simulink model "UPSControl"  (R2025b)
settings: Solver=VariableStepAuto  StartTime=0.0  StopTime=10  FixedStep=Ts  RelTol=1e-3
PostLoadFcn:
  | DataCenterParam;
values from neighbouring files (symbols this model uses):
  generator = struct    [GeneratorParam.m]
  lineInductance = 1e-6    (= 1e-06)    [DataCenterParam.m]    (also in GridParam.m)
  lineResistance = 1e-3    (= 0.001)    [DataCenterParam.m]    (also in GridParam.m)
  loadPower = 5e6    (= 5000000)    [DataCenterParam.m]    (also in LVRT.m; RedundancyAnalysis.m = 10000000)
  machine = struct    [GeneratorParam.m]
  powerTau = 0.005    [DataCenterParam.m]
  Ts = 5e-5    (= 5e-05)    [DataCenterParam.m]    (also in GeneratorParam.m)
  utilizationFactor = 0.45    [DataCenterParam.m]    (also in RedundancyAnalysis.m)
undefined symbols (not defined in the file or in its folder): breaker, ctLimitDelayTime, DiscIntNeverNeededParam, ee_sli_rtmsupport, gcbh, grid, rack, ups
libraries: nesl_utility x96, fl_lib x96, eeGeneralControl x84, ee_lib x80, simulink x68, eeTransforms x30, nesl_utility_internal x16, eeSinusoidalMeasurementV2 x13, slpidlib x12, simulink_extras x12, datacenter_lib x5, batteryecm_lib x4
(part 7 of 13)

== system UPSControl/Server Load/UPS Units/Three UPS Parallel/UPS2/DC-Link/BESS ==
  iPFC : Inport
  Vdc : Inport  Port=2
  iChrg : Inport  Port=3
  vPCC : Inport  Port=4
  Brk : Inport  Port=5
  Battery : batteryecm_lib/Battery  Vnom=400 V  prm_dir=simscape.enum.battery.prm_dir.disabled  R1_dis=5e-2 Ohm  R1_ch=1e-3 Ohm  R1=1e-3 Ohm  prm_AH=simscape.enum.battery.prm_AH.infinite  AH=50 A*hr  V1=11.5 V  AH1=25 A*hr  prm_R2=simscape.enum.battery.prm_R2.disabled  R2=2000 Ohm  Tmeas=298.15 K  charge_measurement_port=simscape.enum.battery.enable.yes  prm_dyn=simscape.enum.battery.prm_dyn.off  Rp1=0.005 Ohm  tau1=30 s  Rp2=0.005 Ohm  tau2=30 s  Rp3=0.005 Ohm  tau3=30 s  Rp4=0.005 Ohm  tau4=30 s  Rp5=0.005 Ohm  tau5=30 s  prm_fade=simscape.enum.battery.prm_fade.disabled  N_fade=100  AH_fade=45 A*hr  R1_fade=2.02 Ohm  R1_ch_fade=2.02 Ohm  V1_fade=10.35 V  prm_age=simscape.enum.battery.prm_age.disabled  prm_age_OCV=simscape.enum.battery.prm_age_OCV.OCV  OCV_age=0.9  SOC_age=60  Tmeas_age=298.15 K  delta_time_age_vec=[0] d  temperature_age_vec=[273] K  OCV_scaling_age=2.2134e6  OCV_offset_age=1.632e6  temp_exp_age=0.515833569 V  t_exp_age=0.75  Vnom_T2=12 V  R1_T2=2.2 Ohm  R1_T2_dis=2.2 Ohm  R1_T2_ch=2.2 Ohm  V1_T2=11.4 V  R2_T2=2200 Ohm  Rp1_T2=0.005 Ohm  tau1_T2=30 s  Rp2_T2=0.005 Ohm  tau2_T2=30 s  Rp3_T2=0.005 Ohm  tau3_T2=30 s  Rp4_T2=0.005 Ohm  tau4_T2=30 s  Rp5_T2=0.005 Ohm  tau5_T2=30 s  Tmeas2=273.15 K  thermal_port=simscape.enum.thermaleffects.omit  thermal_mass=30000 J/K  i_specify=on  i_priority=High  i=0 A  i_nominal_specify=off  i_nominal_value=1  i_nominal_unit=A  v_specify=on  v_priority=None  v=400 V  v_nominal_specify=off  v_nominal_value=1  v_nominal_unit=V  charge_specify=on  charge_priority=None  charge=50 A*hr  charge_nominal_specify=off  charge_nominal_value=1  charge_nominal_unit=A*hr  num_cycles_specify=off  num_cycles_priority=High  num_cycles=0  num_cycles_nominal_specify=off  num_cycles_nominal_value=1  num_cycles_nominal_unit=1  temperature_specify=off  temperature_priority=High  temperature=298.15 K  temperature_nominal_specify=off  temperature_nominal_value=1  temperature_nominal_unit=K
      settings: InternalSimscapePortConfiguration="{\"Bottom\":[],\"Left\":[{\"id\":\"p\",\"label\":\"+\",\"type\":\"foundation.electrical.electrical\"},{\"id\":\"q\",\"label\":\"q\",\"type\":\"output\"}],\"Right\":[{\"id\":\"n\",\"label\":\"-\",\"type\":\"foundation.electrical.electrical\"}],\"Top\":[]}"
  Constant : Constant
  Current Sensor : fl_lib/Electrical/Electrical Sensors/Current Sensor
  Current Sensor1 : fl_lib/Electrical/Electrical Sensors/Current Sensor
  DC-DC Converter Controller : Subsystem
  Delay1 : Delay  DelayLength=1  InitialCondition=400
  Delay2 : Delay  DelayLength=1  InitialCondition=400
  Delay3 : Delay  DelayLength=1  InitialCondition=400
  Electrical Reference2 : fl_lib/Electrical/Electrical Elements/Electrical Reference
  PS-Simulink Converter{,1..3} (4 alike) : nesl_utility/PS-Simulink Converter  PhysicalDomain=network_engine_domain  SubClassName=ps_output  LeftPortType=input  RightPortType=output  PseudoPeriodic=off  Frequencies=[]  VectorFormat=inherit  Unit=inherit  AffineConversion=off
  Simscape Component1 : SimscapeComponentBlock  SourceFile=microgridRenewables.biDirectionalConverter  ComponentPath=microgridRenewables.biDirectionalConverter  ComponentVariants="[\"microgridRenewables.biDirectionalConverter\"]"  ComponentVariantNames="[\"biDirectionalConverter\"]"  ClassName=biDirectionalConverter  SchemaVersion=1  efficiency_option=ee.enum.converters.efficiency.constant  efficiency_fixed=100  i_vec=[0, 2, 5] A  efficiency_vec=[90, 95, 98]  iL_specify=off  iL_priority=High  iL=0 A  iL_nominal_specify=off  iL_nominal_value=1  iL_nominal_unit=A  vc_specify=off  vc_priority=High  vc=0 V  vc_nominal_specify=off  vc_nominal_value=1  vc_nominal_unit=V  i1_specify=off  i1_priority=None  i1=0 A  i1_nominal_specify=off  i1_nominal_value=1  i1_nominal_unit=A  i2_specify=off  i2_priority=None  i2=0 A  i2_nominal_specify=off  i2_nominal_value=1  i2_nominal_unit=A  v1_specify=off  v1_priority=None  v1=0 V  v1_nominal_specify=off  v1_nominal_value=1  v1_nominal_unit=V  v2_specify=off  v2_priority=None  v2=0 V  v2_nominal_specify=off  v2_nominal_value=1  v2_nominal_unit=V
      settings: CopyFcn=simscape.sscblock.internal.componentBlockCallback(gcbh,'COPY')  PreCopyFcn=simscape.sscblock.internal.componentBlockCallback(gcbh,'PRECOPY')  PreDeleteFcn=simscape.sscblock.internal.componentBlockCallback(gcbh,'PREDELETE')  InternalSimscapePortConfiguration="{\"Bottom\":[],\"Left\":[{\"id\":\"Iref\",\"label\":\"Iref\",\"type\":\"input\"},{\"id\":\"p1\",\"label\":\"1+\",\"type\":\"foundation.electrical.electrical\"},{\"id\":\"n1\",\"label\":\"1-\",\"type\":\"foundation.electrical.electrical\"}],\"Right\":[{\"id\":\"p2\",\"label\":\"2+\",\"type\":\"foundation.electrical.electrical\"},{\"id\":\"n2\",\"label\":\"2-\",\"type\":\"foundation.electrical.electrical\"}],\"Top\":[]}"
      mask Type: Bi-directional DC-DC Converter
  Voltage Sensor1 : fl_lib/Electrical/Electrical Sensors/Voltage Sensor
  + : PMIOPort  Side=Left
  - : PMIOPort  Port=2  Side=Right
  Ibatt : Outport
  SOC : Outport  Port=2
  IDCDC : Outport  Port=3
  wires:
  iChrg/1 -> DC-DC Converter Controller/5(iCharge)
  Vdc/1 -> DC-DC Converter Controller/2(Vo)
  Delay1/1 -> DC-DC Converter Controller/3(vBatt)
  iPFC/1 -> DC-DC Converter Controller/4(iPFC)
  Constant/1 -> DC-DC Converter Controller/1(Voref)
  PS-Simulink Converter/1 -> Delay2/1
  Delay2/1 -> Ibatt/1, DC-DC Converter Controller/6(iBatt)
  vPCC/1 -> DC-DC Converter Controller/7(vPCC)
  Brk/1 -> DC-DC Converter Controller/8(Breaker)
  PS-Simulink Converter1/1 -> Delay3/1
  Delay3/1 -> SOC/1
  PS-Simulink Converter2/1 -> Delay1/1
  PS-Simulink Converter3/1 -> IDCDC/1
  connections:
  Electrical Reference2/LConn1 -- Simscape Component1/RConn2 -- Voltage Sensor1/RConn2 -- Battery/RConn1
  Battery/LConn1 -- Current Sensor1/RConn2
  PS-Simulink Converter2/LConn1 -- Voltage Sensor1/RConn1
  -/RConn1 -- Simscape Component1/LConn3
  Current Sensor1/LConn1 -- Simscape Component1/RConn1 -- Voltage Sensor1/LConn1
  DC-DC Converter Controller/RConn1 -- Simscape Component1/LConn1
  PS-Simulink Converter/LConn1 -- Current Sensor1/RConn1
  PS-Simulink Converter1/LConn1 -- Battery/LConn2
  Current Sensor/RConn2 -- Simscape Component1/LConn2
  Current Sensor/LConn1 -- +/RConn1
  PS-Simulink Converter3/LConn1 -- Current Sensor/RConn1

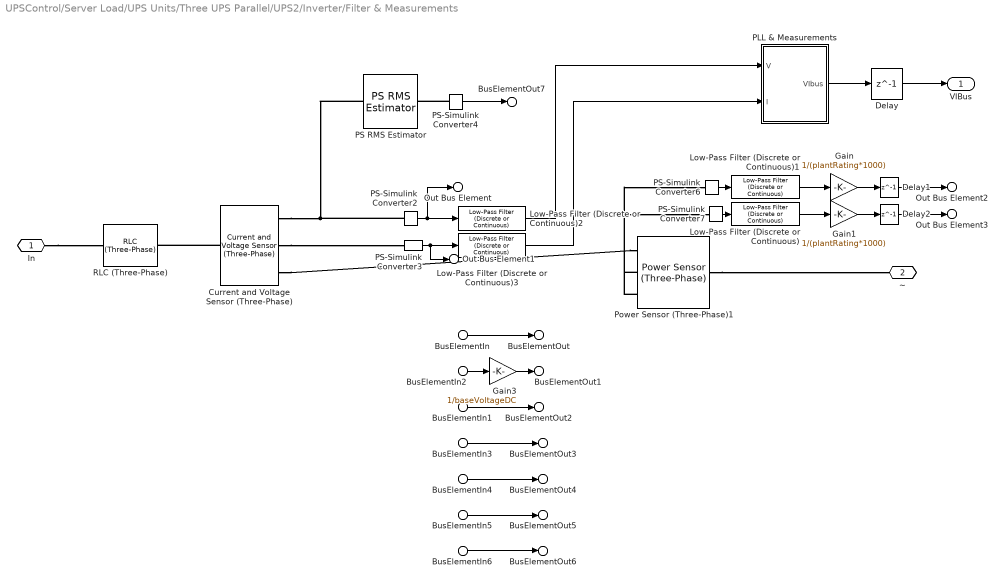
== system UPSControl/Server Load/UPS Units/Three UPS Parallel/UPS2/Inverter/Filter & Measurements ==
  BusElementIn : Inport  PortName=DCBusMeas  Element=SOC
  BusElementIn2 : Inport  PortName=DCBusMeas  Element=Vdc
  BusElementIn1 : Inport  PortName=DCBusMeas  Element=Ibatt
  BusElementIn3 : Inport  PortName=DCBusMeas  Element=Idc
  BusElementIn4 : Inport  PortName=DCBusMeas  Element=ILoad
  BusElementIn5 : Inport  PortName=DCBusMeas  Element=IDCDC
  BusElementIn6 : Inport  PortName=DCBusMeas  Element=UPSBrK
  Current and Voltage Sensor (Three-Phase) : ee_lib/Sensors & Transducers/Current and Voltage Sensor (Three-Phase)  vMeasurementType=ee.enum.vmeasurement.lg  outputUnit=ee.enum.unit.pu  SRated=plantRating*1000 A*V  VRated=Vac V  I_specify=off  I_priority=None  I=[0, 0, 0] A  I_nominal_specify=off  I_nominal_value=1  I_nominal_unit=A  V_specify=off  V_priority=None  V=[0, 0, 0] V  V_nominal_specify=off  V_nominal_value=1  V_nominal_unit=V
      settings: InternalSimscapePortConfiguration="{\"Bottom\":[],\"Left\":[{\"id\":\"N1\",\"label\":\"~1\",\"type\":\"foundation.electrical.three_phase\"}],\"Right\":[{\"id\":\"V_output\",\"label\":\"V\",\"type\":\"output\"},{\"id\":\"I_output\",\"label\":\"I\",\"type\":\"output\"},{\"id\":\"N2\",\"label\":\"~2\",\"type\":\"foundation.electrical.three_phase\"}],\"Top\":[]}"
  Delay : Delay  DelayLength=1
  Delay1 : Delay  DelayLength=1
  Delay2 : Delay  DelayLength=1
  Gain : Gain  Gain=1/(plantRating*1000)
  Gain1 : Gain  Gain=1/(plantRating*1000)
  Gain3 : Gain  Gain=1/baseVoltageDC
  Low-Pass Filter (Discrete or Continuous) : eeGeneralControl/Low-Pass Filter (Discrete or Continuous)  K=1  T=powerTau  B=inf  A=-inf  init_option=Inherited from block input  x0=0  Ts=Ts
  Low-Pass Filter (Discrete or Continuous)1 : eeGeneralControl/Low-Pass Filter (Discrete or Continuous)  K=1  T=powerTau  B=inf  A=-inf  init_option=Inherited from block input  x0=0  Ts=Ts
  Low-Pass Filter (Discrete or Continuous)2 : eeGeneralControl/Low-Pass Filter (Discrete or Continuous)  K=1  T=powerTau/10  B=inf  A=-inf  init_option=Inherited from block input  x0=0  Ts=Ts
  Low-Pass Filter (Discrete or Continuous)3 : eeGeneralControl/Low-Pass Filter (Discrete or Continuous)  K=1  T=powerTau/10  B=inf  A=-inf  init_option=Inherited from block input  x0=0  Ts=Ts
  PLL & Measurements : Subsystem
      mask Display: image('PLL_9_7_2_20_1.png');
  PS RMS Estimator : fl_lib/Physical Signals/Periodic Operators/PS RMS Estimator  f0=60 Hz
      settings: InternalSimscapePortConfiguration="{\"Bottom\":[],\"Left\":[{\"id\":\"I\",\"label\":\"\",\"type\":\"input\"}],\"Right\":[{\"id\":\"O\",\"label\":\"\",\"type\":\"output\"}],\"Top\":[]}"
  PS-Simulink Converter2 : nesl_utility_internal/PS-Simulink Converter  PhysicalDomain=network_engine_domain  SubClassName=ps_output  LeftPortType=input  RightPortType=output  PseudoPeriodic=off  Frequencies=[]  VectorFormat=1-D array  Unit=V  AffineConversion=off
  PS-Simulink Converter3 : nesl_utility_internal/PS-Simulink Converter  PhysicalDomain=network_engine_domain  SubClassName=ps_output  LeftPortType=input  RightPortType=output  PseudoPeriodic=off  Frequencies=[]  VectorFormat=1-D array  Unit=A  AffineConversion=off
  PS-Simulink Converter4 : nesl_utility/PS-Simulink Converter  PhysicalDomain=network_engine_domain  SubClassName=ps_output  LeftPortType=input  RightPortType=output  PseudoPeriodic=off  Frequencies=[]  VectorFormat=inherit  Unit=inherit  AffineConversion=off
  PS-Simulink Converter6 : nesl_utility_internal/PS-Simulink Converter  PhysicalDomain=network_engine_domain  SubClassName=ps_output  LeftPortType=input  RightPortType=output  PseudoPeriodic=off  Frequencies=[]  VectorFormat=1-D array  Unit=W  AffineConversion=off
  PS-Simulink Converter7 : nesl_utility_internal/PS-Simulink Converter  PhysicalDomain=network_engine_domain  SubClassName=ps_output  LeftPortType=input  RightPortType=output  PseudoPeriodic=off  Frequencies=[]  VectorFormat=1-D array  Unit=V*A  AffineConversion=off
  Power Sensor (Three-Phase)1 : ee_lib/Sensors & Transducers/Power Sensor (Three-Phase)  load_type=ee.enum.passive.type_balanced.balanced  f0=60 Hz
      settings: InternalSimscapePortConfiguration="{\"Bottom\":[],\"Left\":[{\"id\":\"N1\",\"label\":\"~1\",\"type\":\"foundation.electrical.three_phase\"}],\"Right\":[{\"id\":\"N2\",\"label\":\"~2\",\"type\":\"foundation.electrical.three_phase\"}],\"Top\":[{\"id\":\"Pm\",\"label\":\"P\",\"type\":\"output\"},{\"id\":\"Qm\",\"label\":\"Q\",\"type\":\"output\"}]}"
  RLC (Three-Phase) : ee_lib/Passive/RLC Assemblies/RLC (Three-Phase)  port_option=ee.enum.threePhasePort.composite  component_structure=ee.enum.rlc.structure.SeriesRL  R=filterResistance %5e-5 Ohm  L=filterInductance%0.00012 H  C=1e-6 F  R_parasitic=0 Ohm  G_parasitic=0 1/Ohm  IL_specify=on  IL_priority=None  IL=[0, 0, 0] A  IL_nominal_specify=off  IL_nominal_value=1  IL_nominal_unit=A  VC_specify=off  VC_priority=High  VC=[0, 0, 0] V  VC_nominal_specify=off  VC_nominal_value=1  VC_nominal_unit=V
      settings: InternalSimscapePortConfiguration="{\"Bottom\":[],\"Left\":[{\"id\":\"N1\",\"label\":\"~1\",\"type\":\"foundation.electrical.three_phase\"}],\"Right\":[{\"id\":\"N2\",\"label\":\"~2\",\"type\":\"foundation.electrical.three_phase\"}],\"Top\":[]}"
  In : PMIOPort  Side=Left
  ~ : PMIOPort  Port=2  Side=Right
  VIBus : Outport
  Out Bus Element : Outport  Port=2  PortName=Meas  Element=voltage
  Out Bus Element1 : Outport  Port=2  PortName=Meas  Element=current
  Out Bus Element2 : Outport  Port=2  PortName=Meas  Element=activePower
  Out Bus Element3 : Outport  Port=2  PortName=Meas  Element=reactivePower
  BusElementOut : Outport  Port=2  PortName=Meas  Element=SOC
  BusElementOut1 : Outport  Port=2  PortName=Meas  Element=Vdc
  BusElementOut2 : Outport  Port=2  PortName=Meas  Element=IBatt
  BusElementOut3 : Outport  Port=2  PortName=Meas  Element=Idc
  BusElementOut4 : Outport  Port=2  PortName=Meas  Element=ILoad
  BusElementOut5 : Outport  Port=2  PortName=Meas  Element=IDCDC
  BusElementOut6 : Outport  Port=2  PortName=Meas  Element=UPSBrK
  BusElementOut7 : Outport  Port=2  PortName=Meas  Element=rmsVoltage
  wires:
  BusElementIn/1 -> BusElementOut/1
  Gain1/1 -> Delay2/1
  Gain/1 -> Delay1/1
  PS-Simulink Converter2/1 -> Out Bus Element/1, Low-Pass Filter (Discrete or Continuous)2/1
  PS-Simulink Converter6/1 -> Low-Pass Filter (Discrete or Continuous)1/1
  PS-Simulink Converter7/1 -> Low-Pass Filter (Discrete or Continuous)/1
  PS-Simulink Converter3/1 -> Out Bus Element1/1, Low-Pass Filter (Discrete or Continuous)3/1
  Low-Pass Filter (Discrete or Continuous)/1 -> Gain1/1
  Low-Pass Filter (Discrete or Continuous)1/1 -> Gain/1
  PLL & Measurements/1(VIbus) -> Delay/1
  Delay/1 -> VIBus/1
  BusElementIn2/1 -> Gain3/1
  Delay1/1 -> Out Bus Element2/1
  Delay2/1 -> Out Bus Element3/1
  BusElementIn1/1 -> BusElementOut2/1
  Gain3/1 -> BusElementOut1/1
  BusElementIn3/1 -> BusElementOut3/1
  BusElementIn4/1 -> BusElementOut4/1
  Low-Pass Filter (Discrete or Continuous)2/1 -> PLL & Measurements/1(V)
  Low-Pass Filter (Discrete or Continuous)3/1 -> PLL & Measurements/2(I)
  BusElementIn5/1 -> BusElementOut5/1
  BusElementIn6/1 -> BusElementOut6/1
  PS-Simulink Converter4/1 -> BusElementOut7/1
  connections:
  Current and Voltage Sensor (Three-Phase)/RConn3 -- Power Sensor (Three-Phase)1/LConn1
  PS-Simulink Converter2/LConn1 -- Current and Voltage Sensor (Three-Phase)/RConn1 -- PS RMS Estimator/LConn1
  Current and Voltage Sensor (Three-Phase)/RConn2 -- PS-Simulink Converter3/LConn1
  Power Sensor (Three-Phase)1/LConn2 -- PS-Simulink Converter6/LConn1
  Power Sensor (Three-Phase)1/LConn3 -- PS-Simulink Converter7/LConn1
  Current and Voltage Sensor (Three-Phase)/LConn1 -- RLC (Three-Phase)/RConn1
  Power Sensor (Three-Phase)1/RConn1 -- ~/RConn1
  In/RConn1 -- RLC (Three-Phase)/LConn1
  PS-Simulink Converter4/LConn1 -- PS RMS Estimator/RConn1

== system UPSControl/Server Load/UPS Units/Three UPS Parallel/UPS2/Inverter/Inverter Controller ==
  VI : Inport
  Power : Inport  Port=2
  Current Limiter : Subsystem
  Droop Control : Subsystem  VariantControl=droop
  VoltageCurrentControl : Subsystem
  mabc : Outport
  wires:
  VI/1 -> VoltageCurrentControl/1(measure), Current Limiter/1(VI)
  VoltageCurrentControl/1(mabc) -> mabc/1
  Droop Control/2(Vqref) -> Current Limiter/3(Vq)
  Droop Control/1(Vdref) -> Current Limiter/2(Vd)
  Droop Control/3(omega) -> VoltageCurrentControl/6(w)
  Droop Control/4(Theta) -> VoltageCurrentControl/7(Angle)
  Current Limiter/3(Idmax) -> VoltageCurrentControl/4(Idmax)
  Current Limiter/2(VqRef) -> VoltageCurrentControl/3(Vqref)
  Current Limiter/1(VdRef) -> VoltageCurrentControl/2(Vdref)
  Current Limiter/4(Iqmax) -> VoltageCurrentControl/5(Iqmax)
  Power/1 -> Droop Control/1(Power)

== system UPSControl/Server Load/UPS Units/Three UPS Parallel/UPS2/Rectifier/Circuit Breaker ==
  BRK : Inport
  Data Type Conversion : DataTypeConversion  OutDataTypeStr=double  SaturateOnIntegerOverflow=off  RndMeth=Floor
  Open Resistance : Gain  Gain=5e7
  Phase Splitter : ee_lib/Connectors & References/Phase Splitter
  Phase Splitter1 : ee_lib/Connectors & References/Phase Splitter
  Simulink-PS Converter : nesl_utility/Simulink-PS Converter  PhysicalDomain=network_engine_domain  SubClassName=ps_input  LeftPortType=input  RightPortType=output  PseudoPeriodic=off  Frequencies=[]  NoiseDistribution=none  NoiseParameters=[]  Unit=1  AffineConversion=off  FilteringAndDerivatives=provide  SimscapeFilterOrder=1  InputFilterTimeConstant=0.001  UdotUserProvided=0
  Variable Resistor : fl_lib/Electrical/Electrical Elements/Variable Resistor  Rmin=1e-3 Ohm  thermalEnable=false  thermal_mass=1 J/K  i_specify=on  i_priority=None  i=0 A  i_nominal_specify=off  i_nominal_value=1  i_nominal_unit=A  v_specify=off  v_priority=None  v=0 V  v_nominal_specify=off  v_nominal_value=1  v_nominal_unit=V  T_specify=off  T_priority=None  T=300 K  T_nominal_specify=off  T_nominal_value=1  T_nominal_unit=K
  Variable Resistor1 : fl_lib/Electrical/Electrical Elements/Variable Resistor  Rmin=1e-3 Ohm  thermalEnable=false  thermal_mass=1 J/K  i_specify=on  i_priority=None  i=0 A  i_nominal_specify=off  i_nominal_value=1  i_nominal_unit=A  v_specify=off  v_priority=None  v=0 V  v_nominal_specify=off  v_nominal_value=1  v_nominal_unit=V  T_specify=off  T_priority=None  T=300 K  T_nominal_specify=off  T_nominal_value=1  T_nominal_unit=K
  Variable Resistor2 : fl_lib/Electrical/Electrical Elements/Variable Resistor  Rmin=1e-3 Ohm  thermalEnable=false  thermal_mass=1 J/K  i_specify=on  i_priority=None  i=0 A  i_nominal_specify=off  i_nominal_value=1  i_nominal_unit=A  v_specify=off  v_priority=None  v=0 V  v_nominal_specify=off  v_nominal_value=1  v_nominal_unit=V  T_specify=off  T_priority=None  T=300 K  T_nominal_specify=off  T_nominal_value=1  T_nominal_unit=K
  ABC2 : PMIOPort  Side=Left
  ~ : PMIOPort  Port=2  Side=Right
  wires:
  Data Type Conversion/1 -> Open Resistance/1
  BRK/1 -> Data Type Conversion/1
  Open Resistance/1 -> Simulink-PS Converter/1
  connections:
  Phase Splitter1/RConn2 -- Variable Resistor1/RConn1
  Variable Resistor1/LConn2 -- Phase Splitter/RConn2
  Phase Splitter1/RConn3 -- Variable Resistor2/RConn1
  Phase Splitter/RConn1 -- Variable Resistor/LConn2
  Variable Resistor2/LConn2 -- Phase Splitter/RConn3
  Phase Splitter1/RConn1 -- Variable Resistor/RConn1
  Phase Splitter1/LConn1 -- ~/RConn1
  Variable Resistor/LConn1 -- Simulink-PS Converter/RConn1 -- Variable Resistor2/LConn1 -- Variable Resistor1/LConn1
  Phase Splitter/LConn1 -- ABC2/RConn1

== system UPSControl/Server Load/UPS Units/Three UPS Parallel/UPS2/Rectifier/Filter & AC measurements ==
  Current : Subsystem
  Current and Voltage Sensor (Three-Phase) : ee_lib/Sensors & Transducers/Current and Voltage Sensor (Three-Phase)  vMeasurementType=ee.enum.vmeasurement.lg  outputUnit=ee.enum.unit.pu  SRated=plantRating*1000 A*V  VRated=Vac V  I_specify=off  I_priority=None  I=[0, 0, 0] A  I_nominal_specify=off  I_nominal_value=1  I_nominal_unit=A  V_specify=off  V_priority=None  V=[0, 0, 0] V  V_nominal_specify=off  V_nominal_value=1  V_nominal_unit=V
      settings: InternalSimscapePortConfiguration="{\"Bottom\":[],\"Left\":[{\"id\":\"N1\",\"label\":\"~1\",\"type\":\"foundation.electrical.three_phase\"}],\"Right\":[{\"id\":\"V_output\",\"label\":\"V\",\"type\":\"output\"},{\"id\":\"I_output\",\"label\":\"I\",\"type\":\"output\"},{\"id\":\"N2\",\"label\":\"~2\",\"type\":\"foundation.electrical.three_phase\"}],\"Top\":[]}"
  Gain : Gain  Gain=1/(plantRating*1000)
  Gain1 : Gain  Gain=1/(plantRating*1000)
  Low-Pass Filter (Discrete or Continuous)1 : eeGeneralControl/Low-Pass Filter (Discrete or Continuous)  K=1  T=10e-3  B=inf  A=-inf  init_option=Inherited from block input  x0=0  Ts=-1
  Low-Pass Filter (Discrete or Continuous)2 : eeGeneralControl/Low-Pass Filter (Discrete or Continuous)  K=1  T=10e-3  B=inf  A=-inf  init_option=Inherited from block input  x0=0  Ts=-1
  PLL : Subsystem
      settings: PortSchema="{\"entries\":[{\"content\":{\"sides\":[{\"content\":{\"connectorIds\":[\"Out1\",\"Out2\",\"Out3\"]},\"type\":\"ConnectorPlacement.EquallySpacedRectSide\",\"uuid\":\"76485780-20fe-4fcf-8224-69648da6ed2a\"},{\"content\":{\"connectorIds\":[\"In1\",\"In2\"],\"side\":\"RIGHT\"},\"type\":\"ConnectorPlacement.EquallySpacedRectSide\",\"uuid\":\"f19a6390-e634-42c7-8d46-4cd80cbab182\"},{\"content\":{\"side\":\"TOP\"},\"type\":\"ConnectorPlacement.EquallySpacedRectSide\",\"uuid\":\"87682f72-1844-428e-be70-ad7ca3191ee3\"}]},\"type\":\"ConnectorPlacement.EquallySpacedConnector\",\"uuid\":\"f2136b07-48ec-402b-adb3-18c0bac2157c\"}],\"packageUris\":[\"http://schema.mathworks.com/mf0/Connector/R2020b\"],\"version\":\"1.0\"}"
  PS-Simulink Converter : nesl_utility/PS-Simulink Converter  PhysicalDomain=network_engine_domain  SubClassName=ps_output  LeftPortType=input  RightPortType=output  PseudoPeriodic=off  Frequencies=[]  VectorFormat=1-D array  Unit=inherit  AffineConversion=off
  PS-Simulink Converter1 : nesl_utility/PS-Simulink Converter  PhysicalDomain=network_engine_domain  SubClassName=ps_output  LeftPortType=input  RightPortType=output  PseudoPeriodic=off  Frequencies=[]  VectorFormat=1-D array  Unit=inherit  AffineConversion=off
  PS-Simulink Converter2 : nesl_utility/PS-Simulink Converter  PhysicalDomain=network_engine_domain  SubClassName=ps_output  LeftPortType=input  RightPortType=output  PseudoPeriodic=off  Frequencies=[]  VectorFormat=inherit  Unit=inherit  AffineConversion=off
  PS-Simulink Converter3 : nesl_utility/PS-Simulink Converter  PhysicalDomain=network_engine_domain  SubClassName=ps_output  LeftPortType=input  RightPortType=output  PseudoPeriodic=off  Frequencies=[]  VectorFormat=inherit  Unit=inherit  AffineConversion=off
  Power Sensor : ee_lib/Sensors & Transducers/Power Sensor (Three-Phase)  load_type=ee.enum.passive.type_balanced.balanced  f0=60 Hz
      settings: InternalSimscapePortConfiguration="{\"Bottom\":[],\"Left\":[{\"id\":\"N1\",\"label\":\"~1\",\"type\":\"foundation.electrical.three_phase\"}],\"Right\":[{\"id\":\"N2\",\"label\":\"~2\",\"type\":\"foundation.electrical.three_phase\"}],\"Top\":[{\"id\":\"Pm\",\"label\":\"P\",\"type\":\"output\"},{\"id\":\"Qm\",\"label\":\"Q\",\"type\":\"output\"}]}"
  RL filter : ee_lib/Passive/RLC Assemblies/RLC (Three-Phase)  port_option=ee.enum.threePhasePort.composite  component_structure=ee.enum.rlc.structure.SeriesRL  R=filterResistanceAFE%0.04 Ohm  L=filterInductanceAFE%6.25e-5 H  C=1e-6 F  R_parasitic=1e-6 Ohm  G_parasitic=1e-6 1/Ohm  IL_specify=on  IL_priority=None  IL=[0, 0, 0] A  IL_nominal_specify=off  IL_nominal_value=1  IL_nominal_unit=A  VC_specify=on  VC_priority=High  VC=[0, 0, 0] V  VC_nominal_specify=off  VC_nominal_value=1  VC_nominal_unit=V
      settings: InternalSimscapePortConfiguration="{\"Bottom\":[],\"Left\":[{\"id\":\"N1\",\"label\":\"~1\",\"type\":\"foundation.electrical.three_phase\"}],\"Right\":[{\"id\":\"N2\",\"label\":\"~2\",\"type\":\"foundation.electrical.three_phase\"}],\"Top\":[]}"
  Voltage : Subsystem
  ABC : PMIOPort  Side=Left
  ABC2 : PMIOPort  Port=2  Side=Right
  Vabc : Outport
  Iabc : Outport  Port=2
  P : Outport  Port=3
  Q : Outport  Port=4
  Id : Outport  Port=5
  freq : Outport  Port=6
  mag : Outport  Port=7
  wires:
  PS-Simulink Converter/1 -> Current/1(Isabc)
  Current/1(Iabc) -> Iabc/1, PLL/1(Iabc)
  PS-Simulink Converter1/1 -> Voltage/1(Vsabc)
  Voltage/1(Vabc) -> Vabc/1, PLL/2(V)
  PS-Simulink Converter2/1 -> Gain/1
  PS-Simulink Converter3/1 -> Gain1/1
  Gain/1 -> Low-Pass Filter (Discrete or Continuous)1/1
  Gain1/1 -> Low-Pass Filter (Discrete or Continuous)2/1
  PLL/1(Id) -> Id/1
  PLL/3(mag) -> mag/1
  PLL/2(freq) -> freq/1
  Low-Pass Filter (Discrete or Continuous)1/1 -> P/1
  Low-Pass Filter (Discrete or Continuous)2/1 -> Q/1
  connections:
  PS-Simulink Converter/LConn1 -- Current and Voltage Sensor (Three-Phase)/RConn2
  PS-Simulink Converter1/LConn1 -- Current and Voltage Sensor (Three-Phase)/RConn1
  Current and Voltage Sensor (Three-Phase)/LConn1 -- ABC/RConn1
  Power Sensor/RConn1 -- RL filter/LConn1
  Power Sensor/LConn1 -- Current and Voltage Sensor (Three-Phase)/RConn3
  PS-Simulink Converter2/LConn1 -- Power Sensor/LConn2
  PS-Simulink Converter3/LConn1 -- Power Sensor/LConn3
  RL filter/RConn1 -- ABC2/RConn1

== system UPSControl/Server Load/UPS Units/Three UPS Parallel/UPS2/Rectifier/PFC Rectifier Controller ==
  VdcRef (V) : Inport
  QRef (pu) : Inport  Port=2
  VdcSens (V) : Inport  Port=3
  VabcSens (pu) : Inport  Port=4
  IabcSens (pu) : Inport  Port=5
  Reset : Inport  Port=6
  Current Controller : Subsystem
  DC Voltage Controller and Current Reference : Subsystem
  PLL : Subsystem
      settings: PortSchema="{\"entries\":[{\"content\":{\"sides\":[{\"content\":{\"connectorIds\":[\"Out1\",\"Out2\",\"Out3\",\"Out4\"]},\"type\":\"ConnectorPlacement.EquallySpacedRectSide\",\"uuid\":\"76485780-20fe-4fcf-8224-69648da6ed2a\"},{\"content\":{\"connectorIds\":[\"In1\"],\"side\":\"RIGHT\"},\"type\":\"ConnectorPlacement.EquallySpacedRectSide\",\"uuid\":\"f19a6390-e634-42c7-8d46-4cd80cbab182\"},{\"content\":{\"side\":\"TOP\"},\"type\":\"ConnectorPlacement.EquallySpacedRectSide\",\"uuid\":\"87682f72-1844-428e-be70-ad7ca3191ee3\"}]},\"type\":\"ConnectorPlacement.EquallySpacedConnector\",\"uuid\":\"f2136b07-48ec-402b-adb3-18c0bac2157c\"}],\"packageUris\":[\"http://schema.mathworks.com/mf0/Connector/R2020b\"],\"version\":\"1.0\"}"
  Rate Transition : RateTransition
  VabcRef (pu) : Outport
  Out Bus Element : Outport  Port=2  PortName=Visualization  Element=pllAngle [rad]
  Out Bus Element1 : Outport  Port=2  PortName=Visualization  Element=pllVmag [pu]
  Out Bus Element2 : Outport  Port=2  PortName=Visualization  Element=Idref [pu]
  Out Bus Element3 : Outport  Port=2  PortName=Visualization  Element=Iqref [pu]
  Out Bus Element5 : Outport  Port=2  PortName=Visualization  Element=IdCntrlError [pu]
  Out Bus Element6 : Outport  Port=2  PortName=Visualization  Element=IqCntrlError [pu]
  wires:
  Current Controller/3(IqCntrlError) -> Out Bus Element6/1
  Current Controller/2(IdCntrlError) -> Out Bus Element5/1
  PLL/1(theta) -> Out Bus Element/1, Current Controller/3(theta)
  Rate Transition/1 -> PLL/1(V)
  DC Voltage Controller and Current Reference/2(iqRef) -> Out Bus Element3/1, Current Controller/2(iqRef)
  DC Voltage Controller and Current Reference/1(idRef) -> Out Bus Element2/1, Current Controller/1(idRef)
  IabcSens (pu)/1 -> Current Controller/6(iabc(PU))
  PLL/3(Vq) -> Current Controller/5(vq)
  PLL/2(Vd) -> Current Controller/4(vd)
  VdcSens (V)/1 -> DC Voltage Controller and Current Reference/4(VdcSens)
  Current Controller/1(vabcRef) -> VabcRef (pu)/1
  PLL/4(mag) -> DC Voltage Controller and Current Reference/2(vPeak), Out Bus Element1/1
  QRef (pu)/1 -> DC Voltage Controller and Current Reference/1(qRef)
  VabcSens (pu)/1 -> Rate Transition/1
  VdcRef (V)/1 -> DC Voltage Controller and Current Reference/3(vdcRef)
  Reset/1 -> Current Controller/7(Reset), DC Voltage Controller and Current Reference/5(Reset)

== system UPSControl/Server Load/UPS Units/Three UPS Parallel/UPS2/Rectifier/Subsystem ==
  In : Inport
  Constant : Constant  Value=0  OutDataTypeStr=boolean
  Delay : Delay  DelayLength=700  SampleTime=ups.sampleTime
  Detect Decrease : simulink/Logic and Bit Operations/Detect Decrease  vinit=0.0  OutDataTypeStr=boolean
  S-R Flip-Flop1 : simulink_extras/Flip Flops/S-R Flip-Flop  initial_condition=0
  Switch : Switch  Criteria=u2 > Threshold  SaturateOnIntegerOverflow=off  InputSameDT=off
  Out : Outport
  wires:
  In/1 -> Detect Decrease/1, Switch/3, Delay/1
  Switch/1 -> Out/1
  Detect Decrease/1 -> S-R Flip-Flop1/1
  Delay/1 -> Switch/1
  S-R Flip-Flop1/1 -> Switch/2
  Constant/1 -> S-R Flip-Flop1/2

== system UPSControl/Server Load/UPS Units/Three UPS Parallel/UPS2/Rectifier/Transfer Control ==
  IBatt : Inport
  Id : Inport  Port=2
  Freq : Inport  Port=3
  Mag : Inport  Port=4
  AND2 : Logic  IconShape=distinctive  AllPortsSameDT=off  OutDataTypeStr=boolean
  AND3 : Logic  IconShape=distinctive  AllPortsSameDT=off  OutDataTypeStr=boolean
  Battery Current Flag : Subsystem
  Data Type Conversion : DataTypeConversion  OutDataTypeStr=boolean  SaturateOnIntegerOverflow=off  RndMeth=Floor
  Frequency Flag : Subsystem
  NOT1 : Logic  Operator=NOT  IconShape=distinctive  AllPortsSameDT=off  OutDataTypeStr=boolean
  NOT2 : Logic  Operator=NOT  IconShape=distinctive  AllPortsSameDT=off  OutDataTypeStr=boolean
  OR : Logic  Operator=OR  IconShape=distinctive  AllPortsSameDT=off  OutDataTypeStr=boolean
  OR1 : Logic  Operator=OR  IconShape=distinctive  AllPortsSameDT=off  OutDataTypeStr=boolean
  PCC Voltage Flag : Subsystem
  PCC Voltage Flag2 : Subsystem
  PFC Current Flag : Subsystem
  S-R Flip-Flop : simulink_extras/Flip Flops/S-R Flip-Flop  initial_condition=0
  S-R Flip-Flop1 : simulink_extras/Flip Flops/S-R Flip-Flop  initial_condition=0
  Step : Step  Time=breaker.grid  SampleTime=0
  Breaker : Outport
  wires:
  PFC Current Flag/1(IdFlag) -> OR/1
  S-R Flip-Flop/1 -> S-R Flip-Flop1/1
  Id/1 -> PFC Current Flag/1(u)
  Mag/1 -> PCC Voltage Flag2/1(u), PCC Voltage Flag/1(u)
  Freq/1 -> Frequency Flag/1(u)
  S-R Flip-Flop1/1 -> Breaker/1
  IBatt/1 -> Battery Current Flag/1(u)
  Frequency Flag/1(FreqFlag) -> AND2/1
  NOT2/1 -> S-R Flip-Flop/2
  Battery Current Flag/1(IBattFlag) -> NOT2/1
  AND2/1 -> S-R Flip-Flop1/2
  OR/1 -> AND3/1
  Step/1 -> Data Type Conversion/1
  AND3/1 -> OR1/2
  Data Type Conversion/1 -> OR1/1
  OR1/1 -> S-R Flip-Flop/1
  PCC Voltage Flag/1(VFlag) -> NOT1/1
  NOT1/1 -> AND2/2
  PCC Voltage Flag2/1(VFlag) -> AND3/2, OR/2

== system UPSControl/Server Load/UPS Units/Three UPS Parallel/UPS3/DC-Link/BESS ==
  iPFC : Inport
  Vdc : Inport  Port=2
  iChrg : Inport  Port=3
  vPCC : Inport  Port=4
  Brk : Inport  Port=5
  Battery : batteryecm_lib/Battery  Vnom=400 V  prm_dir=simscape.enum.battery.prm_dir.disabled  R1_dis=5e-2 Ohm  R1_ch=1e-3 Ohm  R1=1e-3 Ohm  prm_AH=simscape.enum.battery.prm_AH.infinite  AH=50 A*hr  V1=11.5 V  AH1=25 A*hr  prm_R2=simscape.enum.battery.prm_R2.disabled  R2=2000 Ohm  Tmeas=298.15 K  charge_measurement_port=simscape.enum.battery.enable.yes  prm_dyn=simscape.enum.battery.prm_dyn.off  Rp1=0.005 Ohm  tau1=30 s  Rp2=0.005 Ohm  tau2=30 s  Rp3=0.005 Ohm  tau3=30 s  Rp4=0.005 Ohm  tau4=30 s  Rp5=0.005 Ohm  tau5=30 s  prm_fade=simscape.enum.battery.prm_fade.disabled  N_fade=100  AH_fade=45 A*hr  R1_fade=2.02 Ohm  R1_ch_fade=2.02 Ohm  V1_fade=10.35 V  prm_age=simscape.enum.battery.prm_age.disabled  prm_age_OCV=simscape.enum.battery.prm_age_OCV.OCV  OCV_age=0.9  SOC_age=60  Tmeas_age=298.15 K  delta_time_age_vec=[0] d  temperature_age_vec=[273] K  OCV_scaling_age=2.2134e6  OCV_offset_age=1.632e6  temp_exp_age=0.515833569 V  t_exp_age=0.75  Vnom_T2=12 V  R1_T2=2.2 Ohm  R1_T2_dis=2.2 Ohm  R1_T2_ch=2.2 Ohm  V1_T2=11.4 V  R2_T2=2200 Ohm  Rp1_T2=0.005 Ohm  tau1_T2=30 s  Rp2_T2=0.005 Ohm  tau2_T2=30 s  Rp3_T2=0.005 Ohm  tau3_T2=30 s  Rp4_T2=0.005 Ohm  tau4_T2=30 s  Rp5_T2=0.005 Ohm  tau5_T2=30 s  Tmeas2=273.15 K  thermal_port=simscape.enum.thermaleffects.omit  thermal_mass=30000 J/K  i_specify=on  i_priority=High  i=0 A  i_nominal_specify=off  i_nominal_value=1  i_nominal_unit=A  v_specify=on  v_priority=None  v=400 V  v_nominal_specify=off  v_nominal_value=1  v_nominal_unit=V  charge_specify=on  charge_priority=None  charge=50 A*hr  charge_nominal_specify=off  charge_nominal_value=1  charge_nominal_unit=A*hr  num_cycles_specify=off  num_cycles_priority=High  num_cycles=0  num_cycles_nominal_specify=off  num_cycles_nominal_value=1  num_cycles_nominal_unit=1  temperature_specify=off  temperature_priority=High  temperature=298.15 K  temperature_nominal_specify=off  temperature_nominal_value=1  temperature_nominal_unit=K
      settings: InternalSimscapePortConfiguration="{\"Bottom\":[],\"Left\":[{\"id\":\"p\",\"label\":\"+\",\"type\":\"foundation.electrical.electrical\"},{\"id\":\"q\",\"label\":\"q\",\"type\":\"output\"}],\"Right\":[{\"id\":\"n\",\"label\":\"-\",\"type\":\"foundation.electrical.electrical\"}],\"Top\":[]}"
  Constant : Constant
  Current Sensor : fl_lib/Electrical/Electrical Sensors/Current Sensor
  Current Sensor1 : fl_lib/Electrical/Electrical Sensors/Current Sensor
  DC-DC Converter Controller : Subsystem
  Delay1 : Delay  DelayLength=1  InitialCondition=400
  Delay2 : Delay  DelayLength=1  InitialCondition=400
  Delay3 : Delay  DelayLength=1  InitialCondition=400
  Electrical Reference2 : fl_lib/Electrical/Electrical Elements/Electrical Reference
  PS-Simulink Converter{,1..3} (4 alike) : nesl_utility/PS-Simulink Converter  PhysicalDomain=network_engine_domain  SubClassName=ps_output  LeftPortType=input  RightPortType=output  PseudoPeriodic=off  Frequencies=[]  VectorFormat=inherit  Unit=inherit  AffineConversion=off
  Simscape Component1 : SimscapeComponentBlock  SourceFile=microgridRenewables.biDirectionalConverter  ComponentPath=microgridRenewables.biDirectionalConverter  ComponentVariants="[\"microgridRenewables.biDirectionalConverter\"]"  ComponentVariantNames="[\"biDirectionalConverter\"]"  ClassName=biDirectionalConverter  SchemaVersion=1  efficiency_option=ee.enum.converters.efficiency.constant  efficiency_fixed=100  i_vec=[0, 2, 5] A  efficiency_vec=[90, 95, 98]  iL_specify=off  iL_priority=High  iL=0 A  iL_nominal_specify=off  iL_nominal_value=1  iL_nominal_unit=A  vc_specify=off  vc_priority=High  vc=0 V  vc_nominal_specify=off  vc_nominal_value=1  vc_nominal_unit=V  i1_specify=off  i1_priority=None  i1=0 A  i1_nominal_specify=off  i1_nominal_value=1  i1_nominal_unit=A  i2_specify=off  i2_priority=None  i2=0 A  i2_nominal_specify=off  i2_nominal_value=1  i2_nominal_unit=A  v1_specify=off  v1_priority=None  v1=0 V  v1_nominal_specify=off  v1_nominal_value=1  v1_nominal_unit=V  v2_specify=off  v2_priority=None  v2=0 V  v2_nominal_specify=off  v2_nominal_value=1  v2_nominal_unit=V
      settings: CopyFcn=simscape.sscblock.internal.componentBlockCallback(gcbh,'COPY')  PreCopyFcn=simscape.sscblock.internal.componentBlockCallback(gcbh,'PRECOPY')  PreDeleteFcn=simscape.sscblock.internal.componentBlockCallback(gcbh,'PREDELETE')  InternalSimscapePortConfiguration="{\"Bottom\":[],\"Left\":[{\"id\":\"Iref\",\"label\":\"Iref\",\"type\":\"input\"},{\"id\":\"p1\",\"label\":\"1+\",\"type\":\"foundation.electrical.electrical\"},{\"id\":\"n1\",\"label\":\"1-\",\"type\":\"foundation.electrical.electrical\"}],\"Right\":[{\"id\":\"p2\",\"label\":\"2+\",\"type\":\"foundation.electrical.electrical\"},{\"id\":\"n2\",\"label\":\"2-\",\"type\":\"foundation.electrical.electrical\"}],\"Top\":[]}"
      mask Type: Bi-directional DC-DC Converter
  Voltage Sensor1 : fl_lib/Electrical/Electrical Sensors/Voltage Sensor
  + : PMIOPort  Side=Left
  - : PMIOPort  Port=2  Side=Right
  Ibatt : Outport
  SOC : Outport  Port=2
  IDCDC : Outport  Port=3
  wires:
  iChrg/1 -> DC-DC Converter Controller/5(iCharge)
  Vdc/1 -> DC-DC Converter Controller/2(Vo)
  Delay1/1 -> DC-DC Converter Controller/3(vBatt)
  iPFC/1 -> DC-DC Converter Controller/4(iPFC)
  Constant/1 -> DC-DC Converter Controller/1(Voref)
  PS-Simulink Converter/1 -> Delay2/1
  Delay2/1 -> Ibatt/1, DC-DC Converter Controller/6(iBatt)
  vPCC/1 -> DC-DC Converter Controller/7(vPCC)
  Brk/1 -> DC-DC Converter Controller/8(Breaker)
  PS-Simulink Converter1/1 -> Delay3/1
  Delay3/1 -> SOC/1
  PS-Simulink Converter2/1 -> Delay1/1
  PS-Simulink Converter3/1 -> IDCDC/1
  connections:
  Electrical Reference2/LConn1 -- Simscape Component1/RConn2 -- Voltage Sensor1/RConn2 -- Battery/RConn1
  Battery/LConn1 -- Current Sensor1/RConn2
  PS-Simulink Converter2/LConn1 -- Voltage Sensor1/RConn1
  -/RConn1 -- Simscape Component1/LConn3
  Current Sensor1/LConn1 -- Simscape Component1/RConn1 -- Voltage Sensor1/LConn1
  DC-DC Converter Controller/RConn1 -- Simscape Component1/LConn1
  PS-Simulink Converter/LConn1 -- Current Sensor1/RConn1
  PS-Simulink Converter1/LConn1 -- Battery/LConn2
  Current Sensor/RConn2 -- Simscape Component1/LConn2
  Current Sensor/LConn1 -- +/RConn1
  PS-Simulink Converter3/LConn1 -- Current Sensor/RConn1

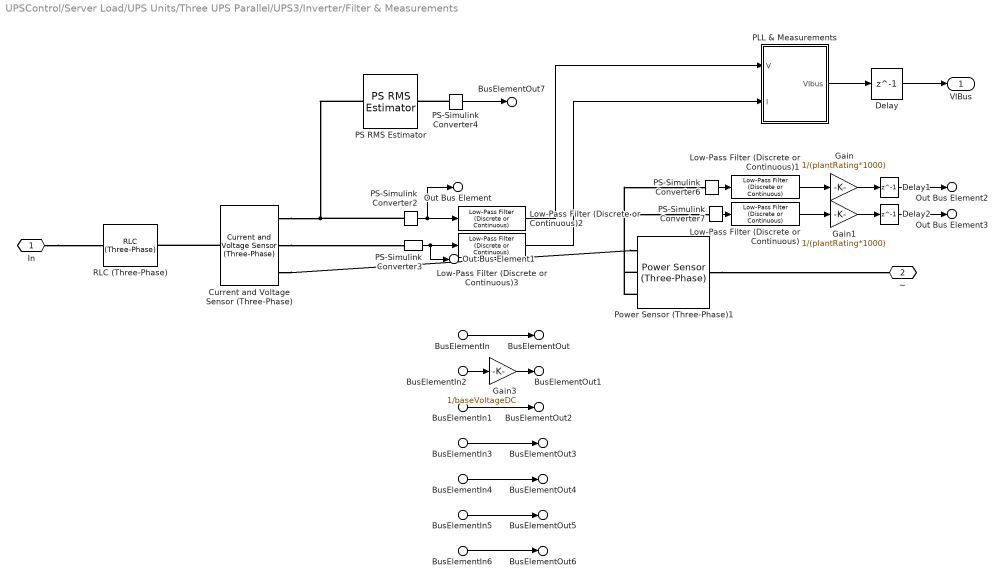
== system UPSControl/Server Load/UPS Units/Three UPS Parallel/UPS3/Inverter/Filter & Measurements ==
  BusElementIn : Inport  PortName=DCBusMeas  Element=SOC
  BusElementIn2 : Inport  PortName=DCBusMeas  Element=Vdc
  BusElementIn1 : Inport  PortName=DCBusMeas  Element=Ibatt
  BusElementIn3 : Inport  PortName=DCBusMeas  Element=Idc
  BusElementIn4 : Inport  PortName=DCBusMeas  Element=ILoad
  BusElementIn5 : Inport  PortName=DCBusMeas  Element=IDCDC
  BusElementIn6 : Inport  PortName=DCBusMeas  Element=UPSBrK
  Current and Voltage Sensor (Three-Phase) : ee_lib/Sensors & Transducers/Current and Voltage Sensor (Three-Phase)  vMeasurementType=ee.enum.vmeasurement.lg  outputUnit=ee.enum.unit.pu  SRated=plantRating*1000 A*V  VRated=Vac V  I_specify=off  I_priority=None  I=[0, 0, 0] A  I_nominal_specify=off  I_nominal_value=1  I_nominal_unit=A  V_specify=off  V_priority=None  V=[0, 0, 0] V  V_nominal_specify=off  V_nominal_value=1  V_nominal_unit=V
      settings: InternalSimscapePortConfiguration="{\"Bottom\":[],\"Left\":[{\"id\":\"N1\",\"label\":\"~1\",\"type\":\"foundation.electrical.three_phase\"}],\"Right\":[{\"id\":\"V_output\",\"label\":\"V\",\"type\":\"output\"},{\"id\":\"I_output\",\"label\":\"I\",\"type\":\"output\"},{\"id\":\"N2\",\"label\":\"~2\",\"type\":\"foundation.electrical.three_phase\"}],\"Top\":[]}"
  Delay : Delay  DelayLength=1
  Delay1 : Delay  DelayLength=1
  Delay2 : Delay  DelayLength=1
  Gain : Gain  Gain=1/(plantRating*1000)
  Gain1 : Gain  Gain=1/(plantRating*1000)
  Gain3 : Gain  Gain=1/baseVoltageDC
  Low-Pass Filter (Discrete or Continuous) : eeGeneralControl/Low-Pass Filter (Discrete or Continuous)  K=1  T=powerTau  B=inf  A=-inf  init_option=Inherited from block input  x0=0  Ts=Ts
  Low-Pass Filter (Discrete or Continuous)1 : eeGeneralControl/Low-Pass Filter (Discrete or Continuous)  K=1  T=powerTau  B=inf  A=-inf  init_option=Inherited from block input  x0=0  Ts=Ts
  Low-Pass Filter (Discrete or Continuous)2 : eeGeneralControl/Low-Pass Filter (Discrete or Continuous)  K=1  T=powerTau/10  B=inf  A=-inf  init_option=Inherited from block input  x0=0  Ts=Ts
  Low-Pass Filter (Discrete or Continuous)3 : eeGeneralControl/Low-Pass Filter (Discrete or Continuous)  K=1  T=powerTau/10  B=inf  A=-inf  init_option=Inherited from block input  x0=0  Ts=Ts
  PLL & Measurements : Subsystem
      mask Display: image('PLL_9_7_2_20_1.png');
  PS RMS Estimator : fl_lib/Physical Signals/Periodic Operators/PS RMS Estimator  f0=60 Hz
      settings: InternalSimscapePortConfiguration="{\"Bottom\":[],\"Left\":[{\"id\":\"I\",\"label\":\"\",\"type\":\"input\"}],\"Right\":[{\"id\":\"O\",\"label\":\"\",\"type\":\"output\"}],\"Top\":[]}"
  PS-Simulink Converter2 : nesl_utility_internal/PS-Simulink Converter  PhysicalDomain=network_engine_domain  SubClassName=ps_output  LeftPortType=input  RightPortType=output  PseudoPeriodic=off  Frequencies=[]  VectorFormat=1-D array  Unit=V  AffineConversion=off
  PS-Simulink Converter3 : nesl_utility_internal/PS-Simulink Converter  PhysicalDomain=network_engine_domain  SubClassName=ps_output  LeftPortType=input  RightPortType=output  PseudoPeriodic=off  Frequencies=[]  VectorFormat=1-D array  Unit=A  AffineConversion=off
  PS-Simulink Converter4 : nesl_utility/PS-Simulink Converter  PhysicalDomain=network_engine_domain  SubClassName=ps_output  LeftPortType=input  RightPortType=output  PseudoPeriodic=off  Frequencies=[]  VectorFormat=inherit  Unit=inherit  AffineConversion=off
  PS-Simulink Converter6 : nesl_utility_internal/PS-Simulink Converter  PhysicalDomain=network_engine_domain  SubClassName=ps_output  LeftPortType=input  RightPortType=output  PseudoPeriodic=off  Frequencies=[]  VectorFormat=1-D array  Unit=W  AffineConversion=off
  PS-Simulink Converter7 : nesl_utility_internal/PS-Simulink Converter  PhysicalDomain=network_engine_domain  SubClassName=ps_output  LeftPortType=input  RightPortType=output  PseudoPeriodic=off  Frequencies=[]  VectorFormat=1-D array  Unit=V*A  AffineConversion=off
  Power Sensor (Three-Phase)1 : ee_lib/Sensors & Transducers/Power Sensor (Three-Phase)  load_type=ee.enum.passive.type_balanced.balanced  f0=60 Hz
      settings: InternalSimscapePortConfiguration="{\"Bottom\":[],\"Left\":[{\"id\":\"N1\",\"label\":\"~1\",\"type\":\"foundation.electrical.three_phase\"}],\"Right\":[{\"id\":\"N2\",\"label\":\"~2\",\"type\":\"foundation.electrical.three_phase\"}],\"Top\":[{\"id\":\"Pm\",\"label\":\"P\",\"type\":\"output\"},{\"id\":\"Qm\",\"label\":\"Q\",\"type\":\"output\"}]}"
  RLC (Three-Phase) : ee_lib/Passive/RLC Assemblies/RLC (Three-Phase)  port_option=ee.enum.threePhasePort.composite  component_structure=ee.enum.rlc.structure.SeriesRL  R=filterResistance %5e-5 Ohm  L=filterInductance%0.00012 H  C=1e-6 F  R_parasitic=0 Ohm  G_parasitic=0 1/Ohm  IL_specify=on  IL_priority=None  IL=[0, 0, 0] A  IL_nominal_specify=off  IL_nominal_value=1  IL_nominal_unit=A  VC_specify=off  VC_priority=High  VC=[0, 0, 0] V  VC_nominal_specify=off  VC_nominal_value=1  VC_nominal_unit=V
      settings: InternalSimscapePortConfiguration="{\"Bottom\":[],\"Left\":[{\"id\":\"N1\",\"label\":\"~1\",\"type\":\"foundation.electrical.three_phase\"}],\"Right\":[{\"id\":\"N2\",\"label\":\"~2\",\"type\":\"foundation.electrical.three_phase\"}],\"Top\":[]}"
  In : PMIOPort  Side=Left
  ~ : PMIOPort  Port=2  Side=Right
  VIBus : Outport
  Out Bus Element : Outport  Port=2  PortName=Meas  Element=voltage
  Out Bus Element1 : Outport  Port=2  PortName=Meas  Element=current
  Out Bus Element2 : Outport  Port=2  PortName=Meas  Element=activePower
  Out Bus Element3 : Outport  Port=2  PortName=Meas  Element=reactivePower
  BusElementOut : Outport  Port=2  PortName=Meas  Element=SOC
  BusElementOut1 : Outport  Port=2  PortName=Meas  Element=Vdc
  BusElementOut2 : Outport  Port=2  PortName=Meas  Element=IBatt
  BusElementOut3 : Outport  Port=2  PortName=Meas  Element=Idc
  BusElementOut4 : Outport  Port=2  PortName=Meas  Element=ILoad
  BusElementOut5 : Outport  Port=2  PortName=Meas  Element=IDCDC
  BusElementOut6 : Outport  Port=2  PortName=Meas  Element=UPSBrK
  BusElementOut7 : Outport  Port=2  PortName=Meas  Element=rmsVoltage
  wires:
  BusElementIn/1 -> BusElementOut/1
  Gain1/1 -> Delay2/1
  Gain/1 -> Delay1/1
  PS-Simulink Converter2/1 -> Out Bus Element/1, Low-Pass Filter (Discrete or Continuous)2/1
  PS-Simulink Converter6/1 -> Low-Pass Filter (Discrete or Continuous)1/1
  PS-Simulink Converter7/1 -> Low-Pass Filter (Discrete or Continuous)/1
  PS-Simulink Converter3/1 -> Out Bus Element1/1, Low-Pass Filter (Discrete or Continuous)3/1
  Low-Pass Filter (Discrete or Continuous)/1 -> Gain1/1
  Low-Pass Filter (Discrete or Continuous)1/1 -> Gain/1
  PLL & Measurements/1(VIbus) -> Delay/1
  Delay/1 -> VIBus/1
  BusElementIn2/1 -> Gain3/1
  Delay1/1 -> Out Bus Element2/1
  Delay2/1 -> Out Bus Element3/1
  BusElementIn1/1 -> BusElementOut2/1
  Gain3/1 -> BusElementOut1/1
  BusElementIn3/1 -> BusElementOut3/1
  BusElementIn4/1 -> BusElementOut4/1
  Low-Pass Filter (Discrete or Continuous)2/1 -> PLL & Measurements/1(V)
  Low-Pass Filter (Discrete or Continuous)3/1 -> PLL & Measurements/2(I)
  BusElementIn5/1 -> BusElementOut5/1
  BusElementIn6/1 -> BusElementOut6/1
  PS-Simulink Converter4/1 -> BusElementOut7/1
  connections:
  Current and Voltage Sensor (Three-Phase)/RConn3 -- Power Sensor (Three-Phase)1/LConn1
  PS-Simulink Converter2/LConn1 -- Current and Voltage Sensor (Three-Phase)/RConn1 -- PS RMS Estimator/LConn1
  Current and Voltage Sensor (Three-Phase)/RConn2 -- PS-Simulink Converter3/LConn1
  Power Sensor (Three-Phase)1/LConn2 -- PS-Simulink Converter6/LConn1
  Power Sensor (Three-Phase)1/LConn3 -- PS-Simulink Converter7/LConn1
  Current and Voltage Sensor (Three-Phase)/LConn1 -- RLC (Three-Phase)/RConn1
  Power Sensor (Three-Phase)1/RConn1 -- ~/RConn1
  In/RConn1 -- RLC (Three-Phase)/LConn1
  PS-Simulink Converter4/LConn1 -- PS RMS Estimator/RConn1

== system UPSControl/Server Load/UPS Units/Three UPS Parallel/UPS3/Inverter/Inverter Controller ==
  VI : Inport
  Power : Inport  Port=2
  Current Limiter : Subsystem
  Droop Control : Subsystem  VariantControl=droop
  VoltageCurrentControl : Subsystem
  mabc : Outport
  wires:
  VI/1 -> VoltageCurrentControl/1(measure), Current Limiter/1(VI)
  VoltageCurrentControl/1(mabc) -> mabc/1
  Droop Control/2(Vqref) -> Current Limiter/3(Vq)
  Droop Control/1(Vdref) -> Current Limiter/2(Vd)
  Droop Control/3(omega) -> VoltageCurrentControl/6(w)
  Droop Control/4(Theta) -> VoltageCurrentControl/7(Angle)
  Current Limiter/3(Idmax) -> VoltageCurrentControl/4(Idmax)
  Current Limiter/2(VqRef) -> VoltageCurrentControl/3(Vqref)
  Current Limiter/1(VdRef) -> VoltageCurrentControl/2(Vdref)
  Current Limiter/4(Iqmax) -> VoltageCurrentControl/5(Iqmax)
  Power/1 -> Droop Control/1(Power)

== system UPSControl/Server Load/UPS Units/Three UPS Parallel/UPS3/Rectifier/Circuit Breaker ==
  BRK : Inport
  Data Type Conversion : DataTypeConversion  OutDataTypeStr=double  SaturateOnIntegerOverflow=off  RndMeth=Floor
  Open Resistance : Gain  Gain=5e7
  Phase Splitter : ee_lib/Connectors & References/Phase Splitter
  Phase Splitter1 : ee_lib/Connectors & References/Phase Splitter
  Simulink-PS Converter : nesl_utility/Simulink-PS Converter  PhysicalDomain=network_engine_domain  SubClassName=ps_input  LeftPortType=input  RightPortType=output  PseudoPeriodic=off  Frequencies=[]  NoiseDistribution=none  NoiseParameters=[]  Unit=1  AffineConversion=off  FilteringAndDerivatives=provide  SimscapeFilterOrder=1  InputFilterTimeConstant=0.001  UdotUserProvided=0
  Variable Resistor : fl_lib/Electrical/Electrical Elements/Variable Resistor  Rmin=1e-3 Ohm  thermalEnable=false  thermal_mass=1 J/K  i_specify=on  i_priority=None  i=0 A  i_nominal_specify=off  i_nominal_value=1  i_nominal_unit=A  v_specify=off  v_priority=None  v=0 V  v_nominal_specify=off  v_nominal_value=1  v_nominal_unit=V  T_specify=off  T_priority=None  T=300 K  T_nominal_specify=off  T_nominal_value=1  T_nominal_unit=K
  Variable Resistor1 : fl_lib/Electrical/Electrical Elements/Variable Resistor  Rmin=1e-3 Ohm  thermalEnable=false  thermal_mass=1 J/K  i_specify=on  i_priority=None  i=0 A  i_nominal_specify=off  i_nominal_value=1  i_nominal_unit=A  v_specify=off  v_priority=None  v=0 V  v_nominal_specify=off  v_nominal_value=1  v_nominal_unit=V  T_specify=off  T_priority=None  T=300 K  T_nominal_specify=off  T_nominal_value=1  T_nominal_unit=K
  Variable Resistor2 : fl_lib/Electrical/Electrical Elements/Variable Resistor  Rmin=1e-3 Ohm  thermalEnable=false  thermal_mass=1 J/K  i_specify=on  i_priority=None  i=0 A  i_nominal_specify=off  i_nominal_value=1  i_nominal_unit=A  v_specify=off  v_priority=None  v=0 V  v_nominal_specify=off  v_nominal_value=1  v_nominal_unit=V  T_specify=off  T_priority=None  T=300 K  T_nominal_specify=off  T_nominal_value=1  T_nominal_unit=K
  ABC2 : PMIOPort  Side=Left
  ~ : PMIOPort  Port=2  Side=Right
  wires:
  Data Type Conversion/1 -> Open Resistance/1
  BRK/1 -> Data Type Conversion/1
  Open Resistance/1 -> Simulink-PS Converter/1
  connections:
  Phase Splitter1/RConn2 -- Variable Resistor1/RConn1
  Variable Resistor1/LConn2 -- Phase Splitter/RConn2
  Phase Splitter1/RConn3 -- Variable Resistor2/RConn1
  Phase Splitter/RConn1 -- Variable Resistor/LConn2
  Variable Resistor2/LConn2 -- Phase Splitter/RConn3
  Phase Splitter1/RConn1 -- Variable Resistor/RConn1
  Phase Splitter1/LConn1 -- ~/RConn1
  Variable Resistor/LConn1 -- Simulink-PS Converter/RConn1 -- Variable Resistor2/LConn1 -- Variable Resistor1/LConn1
  Phase Splitter/LConn1 -- ABC2/RConn1
